simulink model "obs"  (R2024a)
settings: Solver=VariableStepAuto  StartTime=0.0  StopTime=10.0  RelTol=1e-3
settings Model: Creator=pupkinzalupkin  LastModifiedBy=pupkinzalupkin

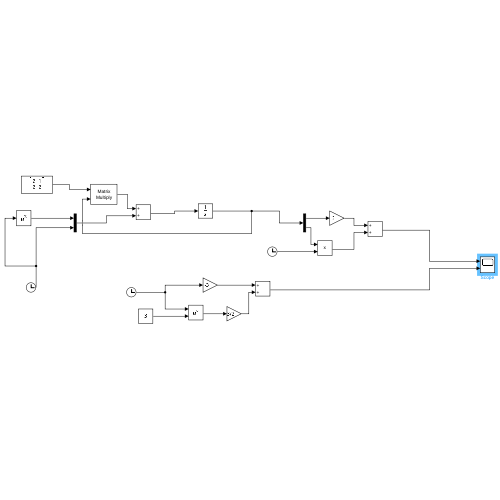
[thumbnail: Simulink's stored preview of the top-level diagram]
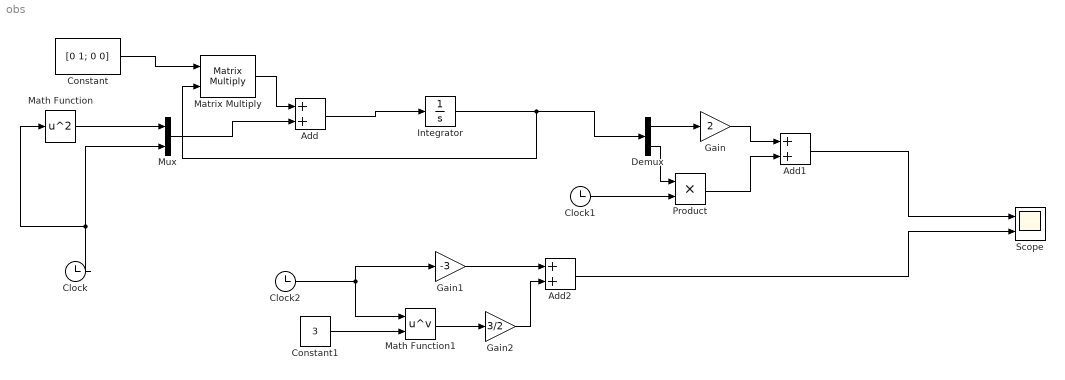
== system obs ==
  Add : Sum
  Add1 : Sum
  Add2 : Sum
  Clock : Clock
  Clock1 : Clock
  Clock2 : Clock
  Constant : Constant  Value=[0 1; 0 0]
  Constant1 : Constant  Value=3
  Demux : Demux  Outputs=2
  Gain : Gain  Gain=2
  Gain1 : Gain  Gain=-3
  Gain2 : Gain  Gain=3/2
  Integrator : Integrator  InitialCondition=[0; -1]
  Math Function : Math  Operator=square
  Math Function1 : Math  Operator=pow
  Matrix Multiply : Product  Multiplication=Matrix(*)
  Mux : Mux  Inputs=2
  Product : Product
  Scope : Scope  NumInputPorts=2
  wires:
  Clock/1 -> Mux/2, Math Function/1
  Math Function/1 -> Mux/1
  Integrator/1 -> Demux/1, Matrix Multiply/2
  Demux/1 -> Gain/1
  Clock1/1 -> Product/2
  Demux/2 -> Product/1
  Gain/1 -> Add1/1
  Product/1 -> Add1/2
  Add1/1 -> Scope/1
  Add2/1 -> Scope/2
  Clock2/1 -> Gain1/1, Math Function1/1
  Gain1/1 -> Add2/1
  Constant1/1 -> Math Function1/2
  Math Function1/1 -> Gain2/1
  Gain2/1 -> Add2/2
  Constant/1 -> Matrix Multiply/1
  Mux/1 -> Add/2
  Matrix Multiply/1 -> Add/1
  Add/1 -> Integrator/1
